simulink model "H_infinity"  (R2018b)
settings: Solver=VariableStepAuto  StartTime=0.0  StopTime=10  RelTol=1e-3
undefined symbols (not defined in the file): den_G, K, num_G
libraries: simulink x1
settings Model: Creator=牟城志  LastModifiedBy=牟城志

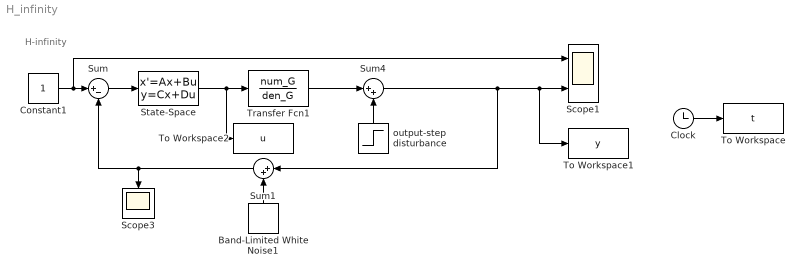
== system H_infinity ==
  note: H-infinity
  Band-Limited White Noise1 : simulink/Sources/Band-Limited White Noise  Cov=1e-7  Ts=1e-3  seed=[23341]
  Clock : Clock
  Constant1 : Constant
  Scope1 : Scope  NumInputPorts=2
  Scope3 : Scope
  State-Space : StateSpace  A=K.A  B=K.B  C=K.C  D=K.D  InitialCondition=0
  Sum : Sum  Inputs=|+-
  Sum1 : Sum  Inputs=|++
  Sum4 : Sum  Inputs=|++
  To Workspace : ToWorkspace  VariableName=t  SampleTime=-1
  To Workspace1 : ToWorkspace  VariableName=y  SampleTime=-1
  To Workspace2 : ToWorkspace  VariableName=u  SampleTime=-1
  Transfer Fcn1 : TransferFcn  Numerator=num_G  Denominator=den_G
  output-step disturbance : Step  Time=4  SampleTime=0
  wires:
  State-Space/1 -> To Workspace2/1, Transfer Fcn1/1
  Constant1/1 -> Scope1/1, Sum/1
  Transfer Fcn1/1 -> Sum4/1
  Sum1/1 -> Sum/2, Scope3/1
  Sum/1 -> State-Space/1
  Sum4/1 -> Sum1/1, To Workspace1/1, Scope1/2
  Clock/1 -> To Workspace/1
  Band-Limited White Noise1/1 -> Sum1/2
  output-step disturbance/1 -> Sum4/2
